simulink model "testecourant"  (R2025a)
settings: Solver=VariableStepAuto  StartTime=0.0  StopTime=5  RelTol=1e-3
undefined symbols (not defined in the file): Acid, Lead
libraries: spsSeriesRLCBranchLib x7, spsDiodeLib x4, spsMosfetLib x4, spsCurrentMeasurementLib x2, spsBatteryLib x1, spsDCVoltageSourceLib x1, spsLinearTransformerLib x1, sps_lib x1
settings Model: Creator=hassan  LastModifiedBy=hassan

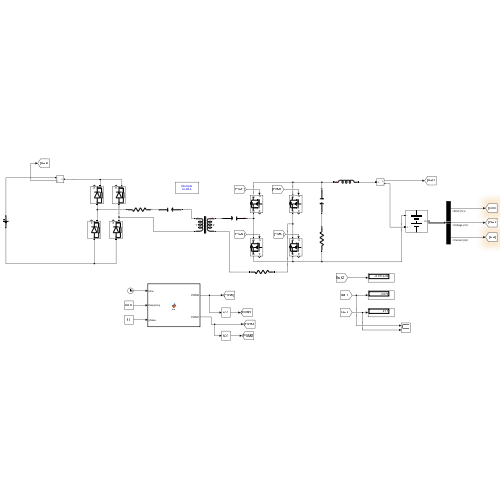
[thumbnail: Simulink's stored preview of the top-level diagram]
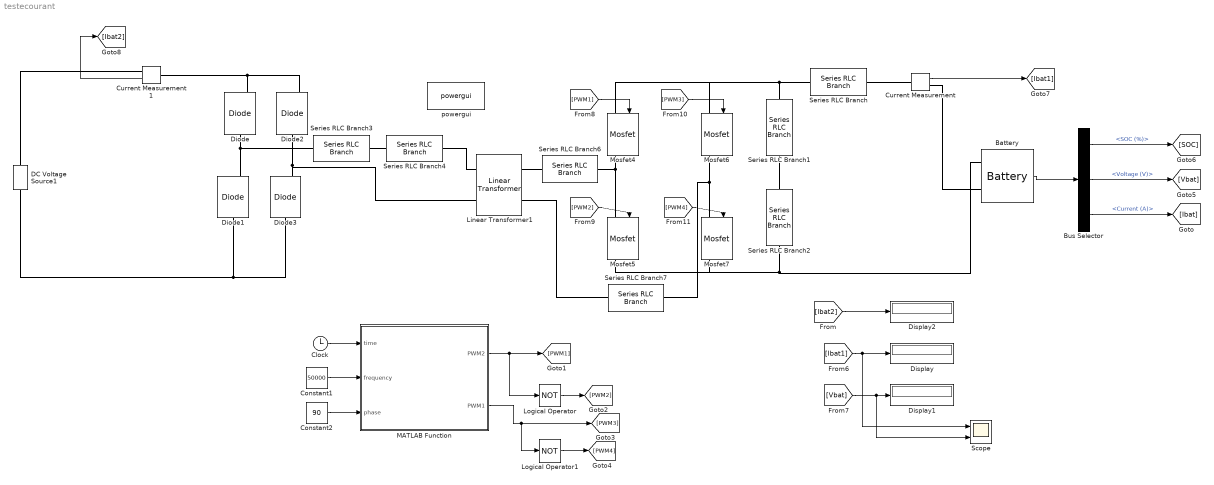
== system testecourant ==
  Battery : spsBatteryLib/Battery  BatType=Lead-Acid  NomV=48  NomQ=150  SOC=50  Batt_Tr=1  PresetModel=on  MaxQ=156.25  MinV=36  FullV=52.2632  Dis_rate=30  R=0.0032  Normal_OP=46.5417  expZone="[48.8684          0.5]"
  Bus Selector : BusSelector  OutputSignals=SOC (%),Voltage (V),Current (A)
  Clock : Clock
  Constant1 : Constant  Value=50000
  Constant2 : Constant  Value=90
  Current Measurement : spsCurrentMeasurementLib/Current Measurement  PhasorSimulation=off  OutputType=Complex  PSBequivalent=0
  Current Measurement1 : spsCurrentMeasurementLib/Current Measurement  PhasorSimulation=off  OutputType=Complex  PSBequivalent=0
  DC Voltage Source1 : spsDCVoltageSourceLib/DC Voltage Source  Amplitude=400  Measurements=None
  Diode{,1..3} (4 alike) : spsDiodeLib/Diode  Ron=0.001  Lon=0  Vf=0.8  IC=0  UseSnubber=0  Rs=500  Cs=250e-9  Measurements=on
  Display : Display
  Display1 : Display
  Display2 : Display
  Linear Transformer1 : spsLinearTransformerLib/Linear Transformer  UNITS=SI  NominalPower=[ 2000 80e3 ]  winding1=[400 4.3218e-9 895e-6]  winding2=[70 0.7938e-9 338e-6]  ThreeWindings=off  winding3=[3.15e+05 0.7938 0.084225]  RmLm=[1.0805e+06 2866]  Measurements=None  DataType=on
  Logical Operator : Logic  Operator=NOT  AllPortsSameDT=off  OutDataTypeStr=boolean
  Logical Operator1 : Logic  Operator=NOT  AllPortsSameDT=off  OutDataTypeStr=boolean
  MATLAB Function : MATLAB Function  TreatAsAtomicUnit=on
  Mosfet{4..7} (4 alike) : spsMosfetLib/Mosfet  Ron=0.1  Lon=0  Rd=0.01  Vfd=0  IC=0  Rs=1e5  Cs=inf  Measurements=on
  Scope : Scope  NumInputPorts=2
      settings: ActiveDisplayYMinimum=-5.8957654723127018  ActiveDisplayYMaximum=12.866449511400653
  Series RLC Branch : spsSeriesRLCBranchLib/Series RLC Branch  LConnTagsString=__new0  RConnTagsString=__new0  BranchType=L  Resistance=1  Inductance=40e-6  SetiL0=off  InitialCurrent=0  Capacitance=1e-6  Setx0=off  InitialVoltage=0  Measurements=None
  Series RLC Branch1 : spsSeriesRLCBranchLib/Series RLC Branch  LConnTagsString=__new0  RConnTagsString=__new0  BranchType=C  Resistance=1  Inductance=1e-3  SetiL0=off  InitialCurrent=0  Capacitance=200e-6  Setx0=off  InitialVoltage=0  Measurements=None
  Series RLC Branch2 : spsSeriesRLCBranchLib/Series RLC Branch  LConnTagsString=__new0  RConnTagsString=__new0  BranchType=R  Resistance=10e-3  Inductance=1e-3  SetiL0=off  InitialCurrent=0  Capacitance=1e-6  Setx0=off  InitialVoltage=0  Measurements=None
  Series RLC Branch3 : spsSeriesRLCBranchLib/Series RLC Branch  LConnTagsString=__new0  RConnTagsString=__new0  BranchType=R  Resistance=340e-3  Inductance=1e-3  SetiL0=off  InitialCurrent=0  Capacitance=1e-6  Setx0=off  InitialVoltage=0  Measurements=None
  Series RLC Branch4 : spsSeriesRLCBranchLib/Series RLC Branch  LConnTagsString=__new0  RConnTagsString=__new0  BranchType=C  Resistance=1  Inductance=1e-3  SetiL0=off  InitialCurrent=0  Capacitance=5.86e-9  Setx0=off  InitialVoltage=0  Measurements=None
  Series RLC Branch6 : spsSeriesRLCBranchLib/Series RLC Branch  LConnTagsString=__new0  RConnTagsString=__new0  BranchType=C  Resistance=1  Inductance=1e-3  SetiL0=off  InitialCurrent=0  Capacitance=15.64e-9  Setx0=off  InitialVoltage=0  Measurements=None
  Series RLC Branch7 : spsSeriesRLCBranchLib/Series RLC Branch  LConnTagsString=__new0  RConnTagsString=__new0  BranchType=R  Resistance=195e-3  Inductance=1e-3  SetiL0=off  InitialCurrent=0  Capacitance=1e-6  Setx0=off  InitialVoltage=0  Measurements=None
  powergui : sps_lib/powergui  Priority=1  SimulationMode=Discrete  SampleTime=1e-8  frequency=60  Iterations=50  frequencyindice=0  Pbase=100e6  ErrMax=1e-4  UnitsV=kV  UnitsW=MW  buscounter=0  FunctionMessages=off  echomessages=off  EnableUseOfTLC=off  CurrentSourceSwitches=off  DisableSnubberDevices=off  DisableRonSwitches=off  DisableVfSwitches=off  DisplayEquations=off  AutomaticDiscreteSolvers=off  SolverType=Tustin/Backward Euler (TBE)  Interpol=off  ExternalGateDelay=off  methode=off  Ts=100  x0status=blocks  SPID=on  SwTol=0  HookPort=off  NonlinearTolerance=1e-4  nMaxIteration=100  ContinueOnMaxIteration=off  RestoreLinks=warning  ResistiveCurrentMeasurement=off  Frange=[0:2:500]  Ylog=off  Xlog=on  ShowGrid=off  save=off  variable=ZData  structure=0  ZoomFFT=off  StartTime=0.0  cycles=1  DisplayStyle=1  fundamental=60  FreqAxis=off  MaxFrequency=1000  frequencyindicesteady=1  RmsSteady=1  display=off
  wires:
  MATLAB Function/2(PWM1) -> Logical Operator1/1, [PWM3]
  [Vbat] -> Scope/2, Display1/1
  Constant1/1 -> MATLAB Function/2(frequency)
  Logical Operator1/1 -> [PWM4]
  Bus Selector/1 -> [SOC]  "<SOC (%)>"
  Battery/1 -> Bus Selector/1
  Bus Selector/3 -> [Ibat]  "<Current (A)>"
  [Ibat1] -> Scope/1, Display/1
  Bus Selector/2 -> [Vbat]  "<Voltage (V)>"
  Logical Operator/1 -> [PWM2]
  MATLAB Function/1(PWM2) -> Logical Operator/1, [PWM1]
  Current Measurement/1 -> [Ibat1]
  Clock/1 -> MATLAB Function/1(time)
  [PWM1] -> Mosfet4/1
  [PWM2] -> Mosfet5/1
  [PWM3] -> Mosfet6/1
  [PWM4] -> Mosfet7/1
  Current Measurement1/1 -> [Ibat2]
  [Ibat2] -> Display2/1
  Constant2/1 -> MATLAB Function/3(phase)
  connections:
  Series RLC Branch/LConn1 -- Mosfet4/LConn1 -- Mosfet6/LConn1 -- Series RLC Branch1/LConn1
  Series RLC Branch2/RConn1 -- Mosfet7/RConn1 -- Mosfet5/RConn1 -- Battery/LConn2
  Diode1/LConn1 -- DC Voltage Source1/LConn1 -- Diode3/LConn1
  Battery/LConn1 -- Current Measurement/RConn1
  Series RLC Branch2/LConn1 -- Series RLC Branch1/RConn1
  Series RLC Branch/RConn1 -- Current Measurement/LConn1
  Mosfet5/LConn1 -- Series RLC Branch6/LConn1 -- Mosfet4/RConn1
  Linear Transformer1/RConn2 -- Series RLC Branch7/RConn1
  Diode1/RConn1 -- Diode/LConn1 -- Series RLC Branch3/RConn1
  Diode3/RConn1 -- Linear Transformer1/LConn2 -- Diode2/LConn1
  Diode2/RConn1 -- Current Measurement1/LConn1 -- Diode/RConn1
  Current Measurement1/RConn1 -- DC Voltage Source1/RConn1
  Linear Transformer1/LConn1 -- Series RLC Branch4/RConn1
  Series RLC Branch4/LConn1 -- Series RLC Branch3/LConn1
  Linear Transformer1/RConn1 -- Series RLC Branch6/RConn1
  Mosfet7/LConn1 -- Mosfet6/RConn1 -- Series RLC Branch7/LConn1

== matlab function testecourant/MATLAB Function ==
  data: time input; PWM2 output; frequency input; phase input; PWM1 output
function [PWM2, PWM1] = fcn (time, frequency, phase)
Tswitching = 1/frequency;
PWM1 =0;
PWM2 =0;
y1 = mod (time, Tswitching) ;
if y1 < Tswitching/2
    PWM1 = 1;
end
t_phi = Tswitching*phase/360;
y2 = mod (time+t_phi, Tswitching) ;
if y2 < Tswitching/2
    PWM2 = 1;
end
